simulink model "Model_Refrigeration_OFF"  (R2022a)
settings: Solver=VariableStepAuto  StartTime=0.0  StopTime=properties_8(15,2)  FixedStep=properties_8(14,2)  MaxStep=properties_8(14,2)  RelTol=1e-3  AbsTol=1e-3
InitFcn:
  | tube_D = 0.02; % [m] Refrigerant tube diameter
  | duct_W = 0.4; % [m] Air duct width
  | house_L = 4.5; % [m] House length
  | house_W = 3; % [m] House width
  | house_H = 2; % [m] House height
  | roof_pitch = 0; % [deg] Roof pitch
undefined symbols (not defined in the file or in its folder): alpha_h_ratio_NE, alpha_h_ratio_NW, alpha_h_ratio_SE, alpha_h_ratio_SW, area_furniture, area_roof, area_wall_exterior_NE, area_wall_exterior_NW, area_wall_exterior_SE, area_wall_exterior_SW, area_window, cp_furniture, cp_roof, cp_wall_exterior_NE, cp_wall_exterior_NW, cp_wall_exterior_SE, cp_wall_exterior_SW, cp_window, hc_furniture_interior, hc_roof_exterior, hc_roof_interior, hc_wall_exterior_NE, hc_wall_exterior_NW, hc_wall_exterior_SE, hc_wall_exterior_SW, hc_wall_interior_NE, hc_wall_interior_NW, hc_wall_interior_SE, hc_wall_interior_SW, hc_window_exterior, hc_window_interior, k_roof, k_wall_NE, k_wall_NW, k_wall_SE, k_wall_SW, k_window, l_roof, mass_furniture, pitch_roof, properties_8, Q_infiltration_latent, Q_infiltration_sensible, Q_latent_occupant_skin, Q_lights, Q_motor, Q_occupant, rho_roof, rho_wall_NE, rho_wall_NW, rho_wall_SE, rho_wall_SW, rho_window, SC, sigbuilder_block, T_env, T_house_init, T_init_furniture, T_set, thicnkess_roof ... (+11)
libraries: fl_lib x59, nesl_utility x15, simulink x1
(part 2 of 2)

== system Model_Refrigeration_OFF/Cooling Loads/Solar Loads Roof and Window/Solar Controller1 ==
  Constant : Constant  Value=properties_8(6,3)
  "High " : Constant  Value=750
  Low : Constant  Value=250
  Medium : Constant  Value=500
  Multiport Switch : MultiPortSwitch  Inputs=5  SaturateOnIntegerOverflow=off  InputSameDT=off
  Solar Load Data Heat Flux Window : Subsystem  Tag=STV Subsys  LoadFcn=sigbuilder_block('load');  StartFcn=sigbuilder_block('start');  StopFcn=sigbuilder_block('stop');  ClipboardFcn=sigbuilder_block('clipboard');  mask(Sigbuilder block){tuvar=[0:10]}
      mask help: Simulink:masks:SigbuilderBlock_MD
      mask init:
      | if ~strcmp(get_param(bdroot(gcbh),'SimulationStatus'),'stopped') tuvar = sigbuilder_block('maskInit'); end
      settings: CopyFcn=sigbuilder_block('copy');  DeleteFcn=sigbuilder_block('delete');  ModelCloseFcn=sigbuilder_block('modelClose');  PreSaveFcn=sigbuilder_block('preSave');  PauseFcn=sigbuilder_block('pause');  ContinueFcn=sigbuilder_block('continue');  NameChangeFcn=sigbuilder_block('namechange');  OpenFcn=sigbuilder_block('open',[440 197.091 394.909 397.818 ]);  CloseFcn=sigbuilder_block('close');
      mask Display: plot(0, 0, 100, 100,[2, 2, 32, 32, 2], [68, 8, 8, 68, 68],[32, 2], [38, 38], [32, 19, 2],[53, 60, 44], [32, 17, 17, 2],[16, 16, 31, 31]);txt = getActiveGroup(gcbh);text(2, 100, txt,'verticalAlignment', 'top');
  Very High : Constant  Value=1000
  Out1 : Outport
  wires:
  Very High/1 -> Multiport Switch/3
  Solar Load Data Heat Flux Window/1(Signal 1) -> Multiport Switch/2
  Multiport Switch/1 -> Out1/1
  Constant/1 -> Multiport Switch/1
  "High "/1 -> Multiport Switch/4
  Medium/1 -> Multiport Switch/5
  Low/1 -> Multiport Switch/6

== system Model_Refrigeration_OFF/Cooling Loads/Solar Loads SE/Solar Controller1 ==
  Constant : Constant  Value=properties_8(2,3)
  "High " : Constant  Value=750
  Low : Constant  Value=250
  Medium : Constant  Value=500
  Multiport Switch : MultiPortSwitch  Inputs=5  SaturateOnIntegerOverflow=off  InputSameDT=off
  Solar Load Data Heat Flux SE : Subsystem  Tag=STV Subsys  LoadFcn=sigbuilder_block('load');  StartFcn=sigbuilder_block('start');  StopFcn=sigbuilder_block('stop');  ClipboardFcn=sigbuilder_block('clipboard');  mask(Sigbuilder block){tuvar=[0:10]}
      mask help: Simulink:masks:SigbuilderBlock_MD
      mask init:
      | if ~strcmp(get_param(bdroot(gcbh),'SimulationStatus'),'stopped') tuvar = sigbuilder_block('maskInit'); end
      settings: CopyFcn=sigbuilder_block('copy');  DeleteFcn=sigbuilder_block('delete');  ModelCloseFcn=sigbuilder_block('modelClose');  PreSaveFcn=sigbuilder_block('preSave');  PauseFcn=sigbuilder_block('pause');  ContinueFcn=sigbuilder_block('continue');  NameChangeFcn=sigbuilder_block('namechange');  OpenFcn=sigbuilder_block('open',[408.6 160.8 395.4 320.4 ]);  CloseFcn=sigbuilder_block('close');
      mask Display: plot(0, 0, 100, 100,[2, 2, 32, 32, 2], [68, 8, 8, 68, 68],[32, 2], [38, 38], [32, 19, 2],[53, 60, 44], [32, 17, 17, 2],[16, 16, 31, 31]);txt = getActiveGroup(gcbh);text(2, 100, txt,'verticalAlignment', 'top');
  Very High : Constant  Value=1000
  Out1 : Outport
  wires:
  Very High/1 -> Multiport Switch/3
  Solar Load Data Heat Flux SE/1(Signal 1) -> Multiport Switch/2
  Multiport Switch/1 -> Out1/1
  Constant/1 -> Multiport Switch/1
  "High "/1 -> Multiport Switch/4
  Medium/1 -> Multiport Switch/5
  Low/1 -> Multiport Switch/6

== system Model_Refrigeration_OFF/Cooling Loads/Solar Loads SW/Solar Controller1 ==
  Constant : Constant  Value=properties_8(5,3)
  "High " : Constant  Value=750
  Low : Constant  Value=250
  Medium : Constant  Value=500
  Multiport Switch : MultiPortSwitch  Inputs=5  SaturateOnIntegerOverflow=off  InputSameDT=off
  Solar Load Data Heat Flux SW : Subsystem  Tag=STV Subsys  LoadFcn=sigbuilder_block('load');  StartFcn=sigbuilder_block('start');  StopFcn=sigbuilder_block('stop');  ClipboardFcn=sigbuilder_block('clipboard');  mask(Sigbuilder block){tuvar=[0:10]}
      mask help: Simulink:masks:SigbuilderBlock_MD
      mask init:
      | if ~strcmp(get_param(bdroot(gcbh),'SimulationStatus'),'stopped') tuvar = sigbuilder_block('maskInit'); end
      settings: CopyFcn=sigbuilder_block('copy');  DeleteFcn=sigbuilder_block('delete');  ModelCloseFcn=sigbuilder_block('modelClose');  PreSaveFcn=sigbuilder_block('preSave');  PauseFcn=sigbuilder_block('pause');  ContinueFcn=sigbuilder_block('continue');  NameChangeFcn=sigbuilder_block('namechange');  OpenFcn=sigbuilder_block('open',[400.8 81.6 395.4 359.4 ]);  CloseFcn=sigbuilder_block('close');
      mask Display: plot(0, 0, 100, 100,[2, 2, 32, 32, 2], [68, 8, 8, 68, 68],[32, 2], [38, 38], [32, 19, 2],[53, 60, 44], [32, 17, 17, 2],[16, 16, 31, 31]);txt = getActiveGroup(gcbh);text(2, 100, txt,'verticalAlignment', 'top');
  Very High : Constant  Value=1000
  Out1 : Outport
  wires:
  Very High/1 -> Multiport Switch/3
  Multiport Switch/1 -> Out1/1
  Constant/1 -> Multiport Switch/1
  "High "/1 -> Multiport Switch/4
  Medium/1 -> Multiport Switch/5
  Low/1 -> Multiport Switch/6
  Solar Load Data Heat Flux SW/1(Signal 1) -> Multiport Switch/2

== system Model_Refrigeration_OFF/Cooling Loads/Solar Loads NE/Solar Controller1/Solar Load Data Heat Flux NE ==
  Demux : Demux  Tag=STV Demux  Outputs=1
      settings: DisplayOption=none
  FromWs : FromWorkspace  Tag=STV FromWs  VariableName=tuvar
      SigBuilderData=|
      | common.afterFinalStr = 'Extrapolate'
      | common.sampleTime = 0
      | dataSet.timeRange = [0 32400]
      | dataSet.name = 'Group 1'
      | sbobj.Groups.Name = 'Group 1'
      | sbobj.Groups.Signals.Name = 'Solar Load NE'
      | sbobj.Groups.Signals.XData = [0 3600 7200 10800 14400 18000 21600 25200 28800 28800 32400]
      | sbobj.Groups.Signals.YData = [540 383 203 144 138 134 126 114 95 96 71]
      | sbobj.Groups.TimeRange = [0 32400]
  Solar Load NE : Outport  Tag=STV Outport
  wires:
  FromWs/1 -> Demux/1
  Demux/1 -> Solar Load NE/1

== system Model_Refrigeration_OFF/Cooling Loads/Solar Loads NW/Solar Controller1/Solar Load Data Heat Flux NW ==
  Demux : Demux  Tag=STV Demux  Outputs=1
      settings: DisplayOption=none
  FromWs : FromWorkspace  Tag=STV FromWs  VariableName=tuvar
      SigBuilderData=|
      | common.afterFinalStr = 'Extrapolate'
      | common.sampleTime = 0
      | dataSet.timeRange = [0 32400]
      | dataSet.name = 'Group 1'
      | sbobj.Groups.Name = 'Group 1'
      | sbobj.Groups.Signals.Name = 'Signal 1'
      | sbobj.Groups.Signals.XData = [0 3600 7200 10800 14400 18000 21600 25200 28800 32400]
      | sbobj.Groups.Signals.YData = [95 114 126 134 138 144 203 383 540 590]
      | sbobj.Groups.TimeRange = [0 32400]
  Signal 1 : Outport  Tag=STV Outport
  wires:
  Demux/1 -> Signal 1/1
  FromWs/1 -> Demux/1

== system Model_Refrigeration_OFF/Cooling Loads/Solar Loads Roof and Window/Solar Controller/Solar Load Data Heat Roof ==
  Demux : Demux  Tag=STV Demux  Outputs=1
      settings: DisplayOption=none
  FromWs : FromWorkspace  Tag=STV FromWs  VariableName=tuvar
      SigBuilderData=|
      | common.afterFinalStr = 'Extrapolate'
      | common.sampleTime = 0
      | dataSet.timeRange = [0 32400]
      | dataSet.name = 'Group 1'
      | sbobj.Groups.Name = 'Group 1'
      | sbobj.Groups.Signals.Name = 'Signal 1'
      | sbobj.Groups.Signals.XData = [0 3600 7200 10800 14400 18000 21600 25200 28800 32400]
      | sbobj.Groups.Signals.YData = [528 702 838 922 949 922 838 702 528 320]
      | sbobj.Groups.TimeRange = [0 32400]
  Signal 1 : Outport  Tag=STV Outport
  wires:
  FromWs/1 -> Demux/1
  Demux/1 -> Signal 1/1

== system Model_Refrigeration_OFF/Cooling Loads/Solar Loads Roof and Window/Solar Controller1/Solar Load Data Heat Flux Window ==
  Demux : Demux  Tag=STV Demux  Outputs=1
      settings: DisplayOption=none
  FromWs : FromWorkspace  Tag=STV FromWs  VariableName=tuvar
      SigBuilderData=|
      | common.afterFinalStr = 'Extrapolate'
      | common.sampleTime = 0
      | dataSet.timeRange = [0 32400]
      | dataSet.name = 'Group 1'
      | sbobj.Groups.Name = 'Group 1'
      | sbobj.Groups.Signals.Name = 'Signal 1'
      | sbobj.Groups.Signals.XData = [0 3600 7200 10800 14400 18000 21600 25200 28800 32400]
      | sbobj.Groups.Signals.YData = [483 811 875 803 647 428 185 48 20 0]
      | sbobj.Groups.TimeRange = [0 32400]
  Signal 1 : Outport  Tag=STV Outport
  wires:
  Demux/1 -> Signal 1/1
  FromWs/1 -> Demux/1

== system Model_Refrigeration_OFF/Cooling Loads/Solar Loads SE/Solar Controller1/Solar Load Data Heat Flux SE ==
  Demux : Demux  Tag=STV Demux  Outputs=1
      settings: DisplayOption=none
  FromWs : FromWorkspace  Tag=STV FromWs  VariableName=tuvar
      SigBuilderData=|
      | common.afterFinalStr = 'Extrapolate'
      | common.sampleTime = 0
      | dataSet.timeRange = [0 32400]
      | dataSet.name = 'Group 1'
      | sbobj.Groups.Name = 'Group 1'
      | sbobj.Groups.Signals.Name = 'Signal 1'
      | sbobj.Groups.Signals.XData = [0 3600 7200 10800 14400 18000 21600 25200 28800 32400]
      | sbobj.Groups.Signals.YData = [580 617 576 460 291 155 131 114 95 71]
      | sbobj.Groups.TimeRange = [0 32400]
  Signal 1 : Outport  Tag=STV Outport
  wires:
  Demux/1 -> Signal 1/1
  FromWs/1 -> Demux/1

== system Model_Refrigeration_OFF/Cooling Loads/Solar Loads SW/Solar Controller1/Solar Load Data Heat Flux SW ==
  Demux : Demux  Tag=STV Demux  Outputs=1
      settings: DisplayOption=none
  FromWs : FromWorkspace  Tag=STV FromWs  VariableName=tuvar
      SigBuilderData=|
      | common.afterFinalStr = 'Extrapolate'
      | common.sampleTime = 0
      | dataSet.timeRange = [0 32400]
      | dataSet.name = 'Group 1'
      | sbobj.Groups.Name = 'Group 1'
      | sbobj.Groups.Signals.Name = 'Signal 1'
      | sbobj.Groups.Signals.XData = [0 3600 7200 10800 14400 18000 21600 25200 28800 32400]
      | sbobj.Groups.Signals.YData = [95 114 131 155 291 460 576 617 580 460]
      | sbobj.Groups.TimeRange = [0 32400]
  Signal 1 : Outport  Tag=STV Outport
  wires:
  FromWs/1 -> Demux/1
  Demux/1 -> Signal 1/1
